simulink model "ASM1"  (R2024b)
settings: Solver=VariableStepAuto  StartTime=0.0  StopTime=100  RelTol=1e-2
values from neighbouring files (symbols this model uses):
  b_A = 0.05    [Input.m]
  b_H = 0.3    [Input.m]
  f_P = 0.08    [Input.m]
  i_X_B = 0.086    [Input.m]
  i_X_P = 0.06    [Input.m]
  k_a = 0.08    [Input.m]
  k_h = 3    [Input.m]
  K_N_H = 1    [Input.m]
  K_N_O = 0.5    [Input.m]
  K_O_A = 0.4    [Input.m]
  K_O_H = 0.2    [Input.m]
  K_S = 20    [Input.m]
  K_X = 0.03    [Input.m]
  mu_A = 0.8    [Input.m]
  mu_H = 6    [Input.m]
  nuy_g = 0.8    [Input.m]
  nuy_h = 0.4    [Input.m]
  Q_1 = 1000    [Input.m]
  Q_2 = Q_1    (= 1000)    [Input.m]
  S_ALK = 5    [Input.m]
  S_I = 40    [Input.m]
  S_ND = 8    [Input.m]
  S_NH = 1    [Input.m]
  S_NO = 0.5    [Input.m]
  S_O = 0.002    [Input.m]
  S_S = 125    [Input.m]
  V_tank = 10000    [Input.m]
  X_B_A = 1    [Input.m]
  X_B_H = 1    [Input.m]
  X_I = 100    [Input.m]
  X_ND = 10    [Input.m]
  X_P = 1    [Input.m]
  X_S = 250    [Input.m]
  Y_A = 0.24    [Input.m]
  Y_H = 0.67    [Input.m]
settings Model: Creator=luima  LastModifiedBy=luima

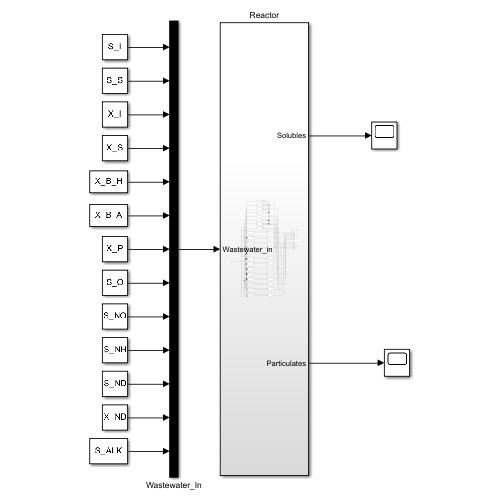
[thumbnail: Simulink's stored preview of the top-level diagram]
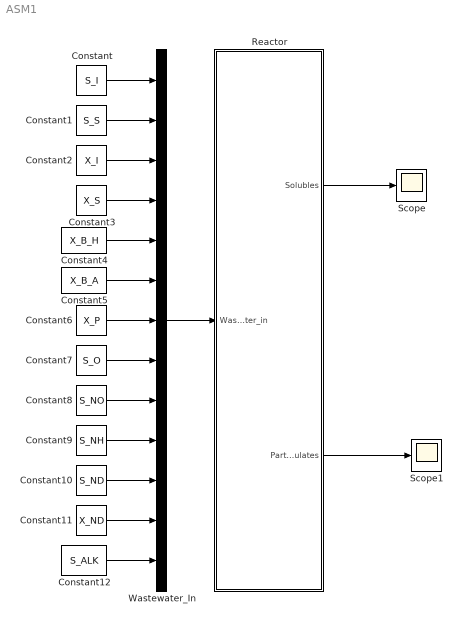
== system ASM1 ==
  Constant : Constant  Value=S_I
  Constant1 : Constant  Value=S_S
  Constant10 : Constant  Value=S_ND
  Constant11 : Constant  Value=X_ND
  Constant12 : Constant  Value=S_ALK
  Constant2 : Constant  Value=X_I
  Constant3 : Constant  Value=X_S
  Constant4 : Constant  Value=X_B_H
  Constant5 : Constant  Value=X_B_A
  Constant6 : Constant  Value=X_P
  Constant7 : Constant  Value=S_O
  Constant8 : Constant  Value=S_NO
  Constant9 : Constant  Value=S_NH
  Reactor : Subsystem
  Scope : Scope
  Scope1 : Scope
  Wastewater_In : Mux  Inputs=13
  wires:
  Constant/1 -> Wastewater_In/1
  Constant1/1 -> Wastewater_In/2
  Constant7/1 -> Wastewater_In/8
  Constant8/1 -> Wastewater_In/9
  Constant9/1 -> Wastewater_In/10
  Constant10/1 -> Wastewater_In/11
  Constant12/1 -> Wastewater_In/13
  Reactor/1(Solubles) -> Scope/1
  Reactor/2(Particulates) -> Scope1/1
  Constant2/1 -> Wastewater_In/3
  Constant3/1 -> Wastewater_In/4
  Constant4/1 -> Wastewater_In/5
  Constant5/1 -> Wastewater_In/6
  Constant6/1 -> Wastewater_In/7
  Constant11/1 -> Wastewater_In/12
  Wastewater_In/1 -> Reactor/1(Wastewater_in)

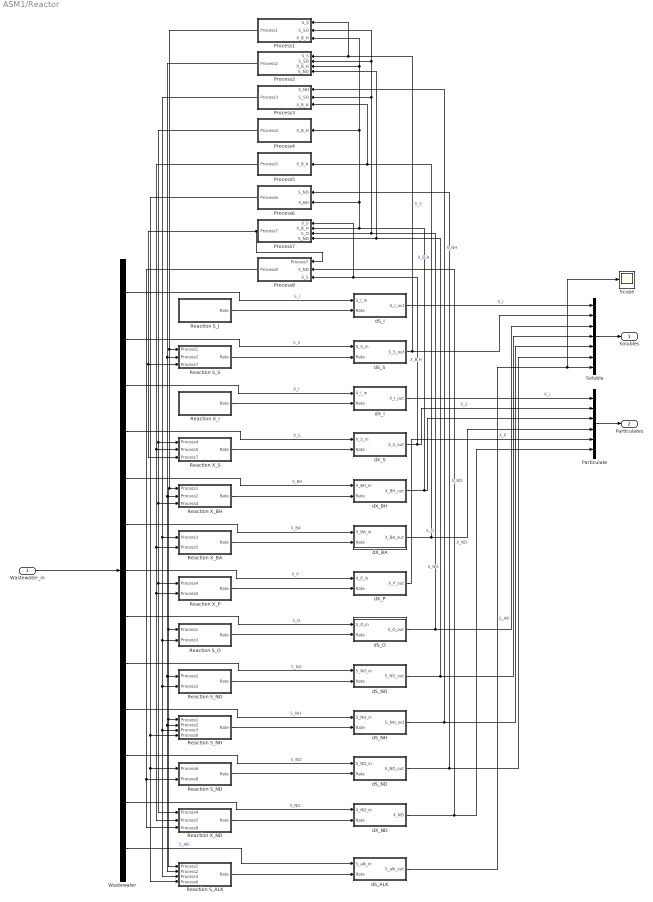
== system ASM1/Reactor ==
  Wastewater_in : Inport
  Particulate : Mux  Inputs=6
  Process1 : Subsystem
  Process2 : Subsystem
  Process3 : Subsystem
  Process4 : Subsystem
  Process5 : Subsystem
  Process6 : Subsystem
  Process7 : Subsystem
  Process8 : Subsystem
  Reaction S_ALK : Subsystem
  Reaction S_I : Subsystem
  Reaction S_ND : Subsystem
  Reaction S_NH : Subsystem
  Reaction S_NO : Subsystem
  Reaction S_O : Subsystem
  Reaction S_S : Subsystem
  Reaction X_BA : Subsystem
  Reaction X_BH : Subsystem
  Reaction X_I : Subsystem
  Reaction X_ND : Subsystem
  Reaction X_P : Subsystem
  Reaction X_S : Subsystem
  Scope : Scope
  Soluble : Mux  Inputs=7
  Wastewater : Demux  Outputs=13
  dS_ALK : Subsystem
  dS_I : Subsystem
  dS_ND : Subsystem
  dS_NH : Subsystem
  dS_NO : Subsystem
  dS_O : Subsystem
  dS_S : Subsystem
  dX_BA : Subsystem
  dX_BH : Subsystem
  dX_I : Subsystem
  dX_ND : Subsystem
  dX_P : Subsystem
  dX_S : Subsystem
  Solubles : Outport
  Particulates : Outport  Port=2
  wires:
  Process7/1(Process7) -> Process8/1(Process7), Reaction S_S/3(Process7), Reaction X_S/3(Process7)
  Process1/1(Process1) -> Reaction S_ALK/1(Process1), Reaction S_NH/1(Process1), Reaction S_O/1(Process1), Reaction X_BH/1(Process1), Reaction S_S/1(Process1)
  Process2/1(Process2) -> Reaction S_ALK/2(Process2), Reaction S_NH/2(Process2), Reaction S_NO/1(Process2), Reaction X_BH/2(Process2), Reaction S_S/2(Process2)
  Process3/1(Process3) -> Reaction X_BA/1(Process3), Reaction S_ALK/3(Process3), Reaction S_NH/3(Process3), Reaction S_NO/2(Process3), Reaction S_O/2(Process3)
  Process4/1(Process4) -> Reaction X_ND/1(Process4), Reaction X_P/1(Process4), Reaction X_BH/3(Process4), Reaction X_S/1(Process4)
  Process5/1(Process5) -> Reaction X_ND/2(Process5), Reaction X_P/2(Process5), Reaction X_BA/2(Process5), Reaction X_S/2(Process5)
  Process6/1(Process6) -> Reaction S_NH/4(Process6), Reaction S_ALK/4(Process6), Reaction S_ND/1(Process6)
  Process8/1(Process8) -> Reaction X_ND/3(Process8), Reaction S_ND/2(Process8)
  Reaction S_I/1(Rate) -> dS_I/2(Rate)
  dS_I/1(S_I_out) -> Soluble/1  "S_I"
  Wastewater/2 -> dS_S/1(S_S_in)  "S_S"
  dS_S/1(S_S_out) -> Process1/1(S_S), Process2/1(S_S), Soluble/2  "S_S"
  Reaction S_S/1(Rate) -> dS_S/2(Rate)
  Wastewater/3 -> dX_I/1(X_I_in)  "X_I"
  dX_I/1(X_I_out) -> Particulate/1  "X_I"
  Reaction X_I/1(Rate) -> dX_I/2(Rate)
  Wastewater/4 -> dX_S/1(X_S_in)  "X_S"
  dX_S/1(X_S_out) -> Process7/1(X_S), Process8/3(X_S), Particulate/2  "X_S"
  Reaction X_S/1(Rate) -> dX_S/2(Rate)
  Wastewater/5 -> dX_BH/1(X_BH_in)  "X_BH"
  Reaction X_BH/1(Rate) -> dX_BH/2(Rate)
  dX_BH/1(X_BH_out) -> Process1/3(X_B_H), Process2/3(X_B_H), Process4/1(X_B_H), Process6/2(X_BH), Process7/2(X_B_H), Particulate/3  "X_B,H"
  Wastewater/6 -> dX_BA/1(X_BA_in)  "X_BA"
  dX_BA/1(X_BA_out) -> Process3/3(X_B_A), Process5/1(X_B_A), Particulate/4  "X_B,A"
  Reaction X_BA/1(Rate) -> dX_BA/2(Rate)
  dX_P/1(X_P_out) -> Particulate/5  "X_P"
  Wastewater/7 -> dX_P/1(X_P_in)  "X_P"
  Reaction X_P/1(Rate) -> dX_P/2(Rate)
  Wastewater/8 -> dS_O/1(S_O_in)  "S_O"
  dS_O/1(S_O_out) -> Process1/2(S_SO), Process2/2(S_SO), Process3/2(S_SO), Process7/3(S_O), Soluble/3  "S_O"
  Reaction S_O/1(Rate) -> dS_O/2(Rate)
  Wastewater/9 -> dS_NO/1(S_NO_in)  "S_NO"
  dS_NO/1(S_NO_out) -> Process2/4(S_NO), Process7/4(S_NO), Soluble/4  "S_NO"
  Reaction S_NO/1(Rate) -> dS_NO/2(Rate)
  Wastewater/10 -> dS_NH/1(S_NH_in)  "S_NH"
  dS_NH/1(S_NH_out) -> Process3/1(S_NH), Soluble/5  "S_NH"
  Reaction S_NH/1(Rate) -> dS_NH/2(Rate)
  Wastewater/11 -> dS_ND/1(S_ND_in)  "S_ND"
  dS_ND/1(S_ND_out) -> Process6/1(S_ND), Soluble/6  "S_ND"
  Reaction S_ND/1(Rate) -> dS_ND/2(Rate)
  Wastewater/12 -> dX_ND/1(X_ND_in)  "X_ND"
  dX_ND/1(X_ND) -> Process8/2(X_ND), Particulate/6  "X_ND"
  Reaction X_ND/1(Rate) -> dX_ND/2(Rate)
  Wastewater/13 -> dS_ALK/1(S_alk_in)  "S_Alk"
  Reaction S_ALK/1(Rate) -> dS_ALK/2(Rate)
  dS_ALK/1(S_alk_out) -> Scope/1, Soluble/7  "S_Alk"
  Wastewater/1 -> dS_I/1(S_I_in)  "S_I"
  Soluble/1 -> Solubles/1
  Particulate/1 -> Particulates/1
  Wastewater_in/1 -> Wastewater/1

== system ASM1/Reactor/Process1 ==
  S_S : Inport
  S_SO : Inport  Port=2
  X_B_H : Inport  Port=3
  A/(A+B) : Subsystem
  A/(A+B)1 : Subsystem
  Constant : Constant  Value=mu_H
  Constant1 : Constant  Value=K_S
  Constant2 : Constant  Value=K_O_H
  Product : Product  Inputs=4
  Process1 : Outport
  wires:
  S_S/1 -> A/(A+B)/1(A)
  Constant1/1 -> A/(A+B)/2(B)
  S_SO/1 -> A/(A+B)1/1(A)
  Constant2/1 -> A/(A+B)1/2(B)
  Constant/1 -> Product/1
  A/(A+B)/1(Out1) -> Product/2
  A/(A+B)1/1(Out1) -> Product/3
  X_B_H/1 -> Product/4
  Product/1 -> Process1/1

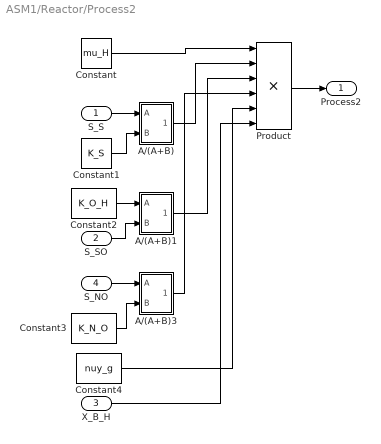
== system ASM1/Reactor/Process2 ==
  S_S : Inport
  S_SO : Inport  Port=2
  X_B_H : Inport  Port=3
  S_NO : Inport  Port=4
  A/(A+B) : Subsystem
  A/(A+B)1 : Subsystem
  A/(A+B)3 : Subsystem
  Constant : Constant  Value=mu_H
  Constant1 : Constant  Value=K_S
  Constant2 : Constant  Value=K_O_H
  Constant3 : Constant  Value=K_N_O
  Constant4 : Constant  Value=nuy_g
  Product : Product  Inputs=6
  Process2 : Outport
  wires:
  S_S/1 -> A/(A+B)/1(A)
  Constant1/1 -> A/(A+B)/2(B)
  Constant/1 -> Product/1
  A/(A+B)/1(Out1) -> Product/2
  A/(A+B)1/1(Out1) -> Product/3
  Constant2/1 -> A/(A+B)1/1(A)
  S_SO/1 -> A/(A+B)1/2(B)
  S_NO/1 -> A/(A+B)3/1(A)
  Constant3/1 -> A/(A+B)3/2(B)
  A/(A+B)3/1(Out1) -> Product/4
  Constant4/1 -> Product/5
  X_B_H/1 -> Product/6
  Product/1 -> Process2/1

== system ASM1/Reactor/Process3 ==
  S_NH : Inport
  S_SO : Inport  Port=2
  X_B_A : Inport  Port=3
  A/(A+B) : Subsystem
  A/(A+B)1 : Subsystem
  Constant : Constant  Value=mu_A
  Constant1 : Constant  Value=K_N_H
  Constant2 : Constant  Value=K_O_A
  Product : Product  Inputs=4
  Process3 : Outport
  wires:
  S_NH/1 -> A/(A+B)/1(A)
  Constant1/1 -> A/(A+B)/2(B)
  S_SO/1 -> A/(A+B)1/1(A)
  Constant2/1 -> A/(A+B)1/2(B)
  Constant/1 -> Product/1
  A/(A+B)/1(Out1) -> Product/2
  A/(A+B)1/1(Out1) -> Product/3
  X_B_A/1 -> Product/4
  Product/1 -> Process3/1

== system ASM1/Reactor/Process4 ==
  X_B_H : Inport
  Constant : Constant  Value=b_H
  Product : Product
  Process4 : Outport
  wires:
  Product/1 -> Process4/1
  Constant/1 -> Product/1
  X_B_H/1 -> Product/2

== system ASM1/Reactor/Process5 ==
  X_B_A : Inport
  Constant : Constant  Value=b_A
  Product : Product
  Process5 : Outport
  wires:
  Product/1 -> Process5/1
  Constant/1 -> Product/1
  X_B_A/1 -> Product/2

== system ASM1/Reactor/Process6 ==
  S_ND : Inport
  X_BH : Inport  Port=2
  Constant : Constant  Value=k_a
  Product : Product  Inputs=3
  Process6 : Outport
  wires:
  Product/1 -> Process6/1
  Constant/1 -> Product/1
  S_ND/1 -> Product/2
  X_BH/1 -> Product/3

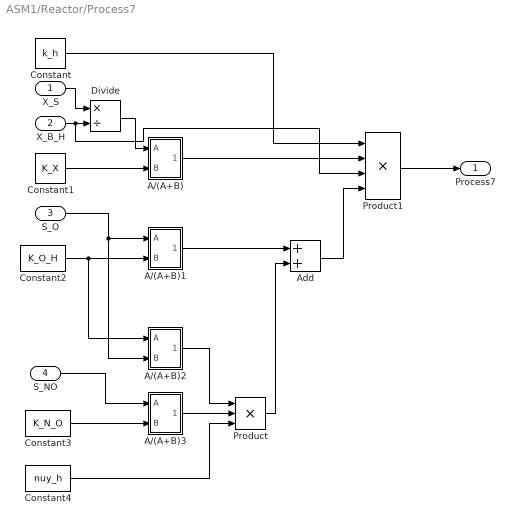
== system ASM1/Reactor/Process7 ==
  X_S : Inport
  X_B_H : Inport  Port=2
  S_O : Inport  Port=3
  S_NO : Inport  Port=4
  A/(A+B) : Subsystem
  A/(A+B)1 : Subsystem
  A/(A+B)2 : Subsystem
  A/(A+B)3 : Subsystem
  Add : Sum
  Constant : Constant  Value=k_h
  Constant1 : Constant  Value=K_X
  Constant2 : Constant  Value=K_O_H
  Constant3 : Constant  Value=K_N_O
  Constant4 : Constant  Value=nuy_h
  Divide : Product  Inputs=*/
  Product : Product  Inputs=3
  Product1 : Product  Inputs=4
  Process7 : Outport
  wires:
  X_S/1 -> Divide/1
  Constant1/1 -> A/(A+B)/2(B)
  Divide/1 -> A/(A+B)/1(A)
  Constant2/1 -> A/(A+B)2/1(A), A/(A+B)1/2(B)
  S_O/1 -> A/(A+B)2/2(B), A/(A+B)1/1(A)
  Constant3/1 -> A/(A+B)3/2(B)
  S_NO/1 -> A/(A+B)3/1(A)
  A/(A+B)3/1(Out1) -> Product/2
  Constant4/1 -> Product/3
  A/(A+B)2/1(Out1) -> Product/1
  Product/1 -> Add/2
  A/(A+B)1/1(Out1) -> Add/1
  Constant/1 -> Product1/1
  A/(A+B)/1(Out1) -> Product1/2
  Add/1 -> Product1/4
  Product1/1 -> Process7/1
  X_B_H/1 -> Product1/3, Divide/2

== system ASM1/Reactor/Process8 ==
  Process7 : Inport
  X_ND : Inport  Port=2
  X_S : Inport  Port=3
  Divide : Product  Inputs=**
  Divide1 : Product  Inputs=*/
  Process8 : Outport
  wires:
  X_ND/1 -> Divide1/1
  X_S/1 -> Divide1/2
  Divide1/1 -> Divide/2
  Process7/1 -> Divide/1
  Divide/1 -> Process8/1

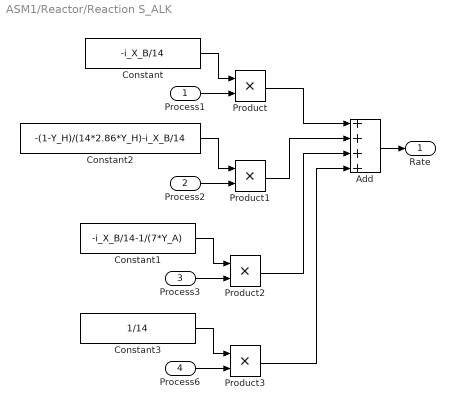
== system ASM1/Reactor/Reaction S_ALK ==
  Process1 : Inport
  Process2 : Inport  Port=2
  Process3 : Inport  Port=3
  Process6 : Inport  Port=4
  Add : Sum  Inputs=++++
  Constant : Constant  Value=-i_X_B/14
  Constant1 : Constant  Value=-i_X_B/14-1/(7*Y_A)
  Constant2 : Constant  Value=-(1-Y_H)/(14*2.86*Y_H)-i_X_B/14
  Constant3 : Constant  Value=1/14
  Product{,1..3} (4 alike) : Product
  Rate : Outport
  wires:
  Process1/1 -> Product/2
  Constant/1 -> Product/1
  Process2/1 -> Product1/2
  Constant2/1 -> Product1/1
  Product/1 -> Add/1
  Product1/1 -> Add/2
  Add/1 -> Rate/1
  Constant1/1 -> Product2/1
  Product2/1 -> Add/3
  Process3/1 -> Product2/2
  Process6/1 -> Product3/2
  Product3/1 -> Add/4
  Constant3/1 -> Product3/1

== system ASM1/Reactor/Reaction S_I ==
  Constant : Constant  Value=0
  Rate : Outport
  wires:
  Constant/1 -> Rate/1

== system ASM1/Reactor/Reaction S_ND ==
  Process6 : Inport
  Process8 : Inport  Port=2
  Add : Sum  Inputs=-+
  Rate : Outport
  wires:
  Process8/1 -> Add/2
  Process6/1 -> Add/1
  Add/1 -> Rate/1

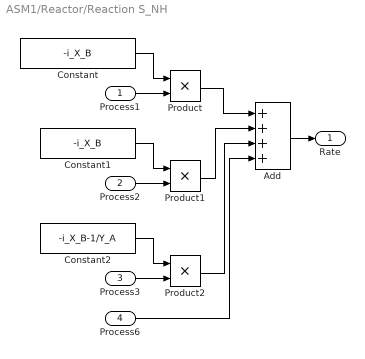
== system ASM1/Reactor/Reaction S_NH ==
  Process1 : Inport
  Process2 : Inport  Port=2
  Process3 : Inport  Port=3
  Process6 : Inport  Port=4
  Add : Sum  Inputs=++++
  Constant : Constant  Value=-i_X_B
  Constant1 : Constant  Value=-i_X_B
  Constant2 : Constant  Value=-i_X_B-1/Y_A
  Product : Product
  Product1 : Product
  Product2 : Product
  Rate : Outport
  wires:
  Process1/1 -> Product/2
  Constant/1 -> Product/1
  Process2/1 -> Product1/2
  Constant1/1 -> Product1/1
  Product/1 -> Add/1
  Product1/1 -> Add/2
  Add/1 -> Rate/1
  Process3/1 -> Product2/2
  Constant2/1 -> Product2/1
  Product2/1 -> Add/3
  Process6/1 -> Add/4

== system ASM1/Reactor/Reaction S_NO ==
  Process2 : Inport
  Process3 : Inport  Port=2
  Add : Sum
  Constant : Constant  Value=-(1-Y_H)/(2.86*Y_H)
  Constant1 : Constant  Value=1/Y_A
  Product : Product
  Product1 : Product
  Rate : Outport
  wires:
  Process2/1 -> Product/2
  Constant/1 -> Product/1
  Process3/1 -> Product1/2
  Constant1/1 -> Product1/1
  Product/1 -> Add/1
  Product1/1 -> Add/2
  Add/1 -> Rate/1

== system ASM1/Reactor/Reaction S_O ==
  Process1 : Inport
  Process3 : Inport  Port=2
  Add : Sum
  Constant : Constant  Value=-(1-Y_H)/Y_H
  Constant1 : Constant  Value=-(4.57-Y_A)/Y_A
  Product : Product
  Product1 : Product
  Rate : Outport
  wires:
  Process1/1 -> Product/2
  Constant/1 -> Product/1
  Process3/1 -> Product1/2
  Constant1/1 -> Product1/1
  Product/1 -> Add/1
  Product1/1 -> Add/2
  Add/1 -> Rate/1

== system ASM1/Reactor/Reaction S_S ==
  Process1 : Inport
  Process2 : Inport  Port=2
  Process7 : Inport  Port=3
  Add : Sum  Inputs=--
  Add1 : Sum
  Constant : Constant  Value=Y_H
  Divide : Product  Inputs=*/
  Rate : Outport
  wires:
  Process1/1 -> Add/1
  Process2/1 -> Add/2
  Constant/1 -> Divide/2
  Add/1 -> Divide/1
  Process7/1 -> Add1/2
  Divide/1 -> Add1/1
  Add1/1 -> Rate/1

== system ASM1/Reactor/Reaction X_BA ==
  Process3 : Inport
  Process5 : Inport  Port=2
  Add : Sum  Inputs=+-
  Rate : Outport
  wires:
  Process5/1 -> Add/2
  Process3/1 -> Add/1
  Add/1 -> Rate/1

== system ASM1/Reactor/Reaction X_BH ==
  Process1 : Inport
  Process2 : Inport  Port=2
  Process4 : Inport  Port=3
  Add : Sum  Inputs=++-
  Rate : Outport
  wires:
  Process2/1 -> Add/2
  Process1/1 -> Add/1
  Process4/1 -> Add/3
  Add/1 -> Rate/1

== system ASM1/Reactor/Reaction X_I ==
  Constant : Constant  Value=0
  Rate : Outport
  wires:
  Constant/1 -> Rate/1

== system ASM1/Reactor/Reaction X_ND ==
  Process4 : Inport
  Process5 : Inport  Port=2
  Process8 : Inport  Port=3
  Add : Sum  Inputs=++-
  Constant : Constant  Value=i_X_B-f_P*i_X_P
  Constant2 : Constant  Value=i_X_B-f_P*i_X_P
  Product : Product
  Product1 : Product
  Rate : Outport
  wires:
  Process4/1 -> Product/2
  Constant/1 -> Product/1
  Process5/1 -> Product1/2
  Constant2/1 -> Product1/1
  Product/1 -> Add/1
  Product1/1 -> Add/2
  Add/1 -> Rate/1
  Process8/1 -> Add/3

== system ASM1/Reactor/Reaction X_P ==
  Process4 : Inport
  Process5 : Inport  Port=2
  Add : Sum
  Constant : Constant  Value=f_P
  Product : Product
  Rate : Outport
  wires:
  Process5/1 -> Add/2
  Process4/1 -> Add/1
  Constant/1 -> Product/2
  Add/1 -> Product/1
  Product/1 -> Rate/1

== system ASM1/Reactor/Reaction X_S ==
  Process4 : Inport
  Process5 : Inport  Port=2
  Process7 : Inport  Port=3
  Add : Sum
  Constant : Constant  Value=1-f_P
  Product : Product
  Subtract : Sum  Inputs=+-
  Rate : Outport
  wires:
  Process5/1 -> Add/2
  Process4/1 -> Add/1
  Constant/1 -> Product/2
  Add/1 -> Product/1
  Process7/1 -> Subtract/2
  Product/1 -> Subtract/1
  Subtract/1 -> Rate/1

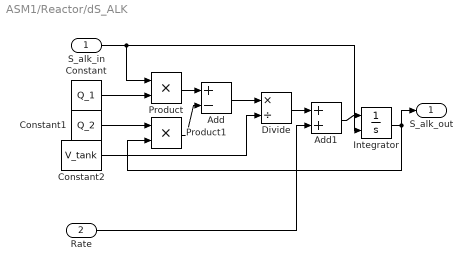
== system ASM1/Reactor/dS_ALK ==
  S_alk_in : Inport
  Rate : Inport  Port=2
  Add : Sum  Inputs=+-
  Add1 : Sum
  Constant : Constant  Value=Q_1
  Constant1 : Constant  Value=Q_2
  Constant2 : Constant  Value=V_tank
  Divide : Product  Inputs=*/
  Integrator : Integrator  InitialConditionSource=external
  Product : Product
  Product1 : Product
  S_alk_out : Outport
  wires:
  Constant/1 -> Product/2
  S_alk_in/1 -> Integrator/2, Product/1
  Integrator/1 -> S_alk_out/1, Product1/2
  Constant1/1 -> Product1/1
  Product/1 -> Add/1
  Product1/1 -> Add/2
  Constant2/1 -> Divide/2
  Add/1 -> Divide/1
  Rate/1 -> Add1/2
  Add1/1 -> Integrator/1
  Divide/1 -> Add1/1

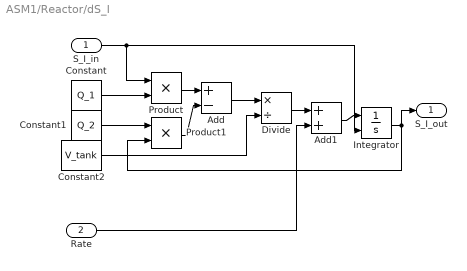
== system ASM1/Reactor/dS_I ==
  S_I_in : Inport
  Rate : Inport  Port=2
  Add : Sum  Inputs=+-
  Add1 : Sum
  Constant : Constant  Value=Q_1
  Constant1 : Constant  Value=Q_2
  Constant2 : Constant  Value=V_tank
  Divide : Product  Inputs=*/
  Integrator : Integrator  InitialConditionSource=external
  Product : Product
  Product1 : Product
  S_I_out : Outport
  wires:
  Constant/1 -> Product/2
  S_I_in/1 -> Integrator/2, Product/1
  Integrator/1 -> S_I_out/1, Product1/2
  Constant1/1 -> Product1/1
  Product/1 -> Add/1
  Product1/1 -> Add/2
  Constant2/1 -> Divide/2
  Add/1 -> Divide/1
  Add1/1 -> Integrator/1
  Divide/1 -> Add1/1
  Rate/1 -> Add1/2

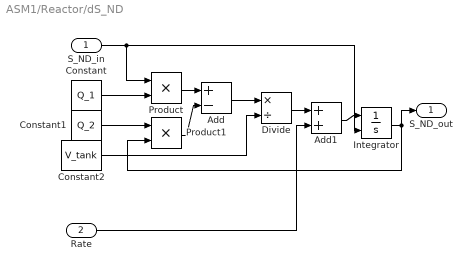
== system ASM1/Reactor/dS_ND ==
  S_ND_in : Inport
  Rate : Inport  Port=2
  Add : Sum  Inputs=+-
  Add1 : Sum
  Constant : Constant  Value=Q_1
  Constant1 : Constant  Value=Q_2
  Constant2 : Constant  Value=V_tank
  Divide : Product  Inputs=*/
  Integrator : Integrator  InitialConditionSource=external
  Product : Product
  Product1 : Product
  S_ND_out : Outport
  wires:
  Constant/1 -> Product/2
  S_ND_in/1 -> Integrator/2, Product/1
  Integrator/1 -> S_ND_out/1, Product1/2
  Constant1/1 -> Product1/1
  Product/1 -> Add/1
  Product1/1 -> Add/2
  Constant2/1 -> Divide/2
  Add/1 -> Divide/1
  Rate/1 -> Add1/2
  Add1/1 -> Integrator/1
  Divide/1 -> Add1/1

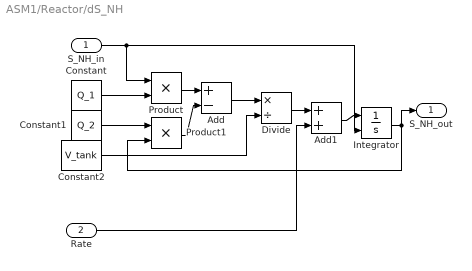
== system ASM1/Reactor/dS_NH ==
  S_NH_in : Inport
  Rate : Inport  Port=2
  Add : Sum  Inputs=+-
  Add1 : Sum
  Constant : Constant  Value=Q_1
  Constant1 : Constant  Value=Q_2
  Constant2 : Constant  Value=V_tank
  Divide : Product  Inputs=*/
  Integrator : Integrator  InitialConditionSource=external
  Product : Product
  Product1 : Product
  S_NH_out : Outport
  wires:
  Constant/1 -> Product/2
  S_NH_in/1 -> Integrator/2, Product/1
  Integrator/1 -> S_NH_out/1, Product1/2
  Constant1/1 -> Product1/1
  Product/1 -> Add/1
  Product1/1 -> Add/2
  Constant2/1 -> Divide/2
  Add/1 -> Divide/1
  Rate/1 -> Add1/2
  Add1/1 -> Integrator/1
  Divide/1 -> Add1/1

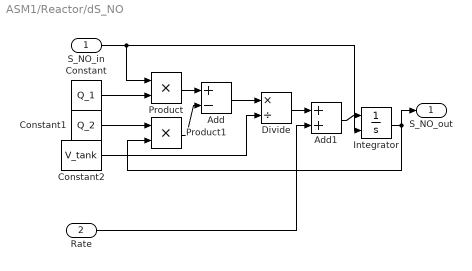
== system ASM1/Reactor/dS_NO ==
  S_NO_in : Inport
  Rate : Inport  Port=2
  Add : Sum  Inputs=+-
  Add1 : Sum
  Constant : Constant  Value=Q_1
  Constant1 : Constant  Value=Q_2
  Constant2 : Constant  Value=V_tank
  Divide : Product  Inputs=*/
  Integrator : Integrator  InitialConditionSource=external
  Product : Product
  Product1 : Product
  S_NO_out : Outport
  wires:
  Constant/1 -> Product/2
  S_NO_in/1 -> Integrator/2, Product/1
  Integrator/1 -> S_NO_out/1, Product1/2
  Constant1/1 -> Product1/1
  Product/1 -> Add/1
  Product1/1 -> Add/2
  Constant2/1 -> Divide/2
  Add/1 -> Divide/1
  Rate/1 -> Add1/2
  Add1/1 -> Integrator/1
  Divide/1 -> Add1/1

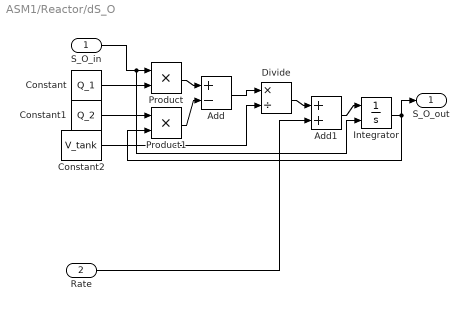
== system ASM1/Reactor/dS_O ==
  S_O_in : Inport
  Rate : Inport  Port=2
  Add : Sum  Inputs=+-
  Add1 : Sum
  Constant : Constant  Value=Q_1
  Constant1 : Constant  Value=Q_2
  Constant2 : Constant  Value=V_tank
  Divide : Product  Inputs=*/
  Integrator : Integrator  InitialConditionSource=external
  Product : Product
  Product1 : Product
  S_O_out : Outport
  wires:
  Constant/1 -> Product/2
  Integrator/1 -> S_O_out/1, Product1/2
  Constant1/1 -> Product1/1
  Product/1 -> Add/1
  Product1/1 -> Add/2
  Constant2/1 -> Divide/2
  Add/1 -> Divide/1
  Rate/1 -> Add1/2
  Add1/1 -> Integrator/1
  Divide/1 -> Add1/1
  S_O_in/1 -> Integrator/2, Product/1

== system ASM1/Reactor/dS_S ==
  S_S_in : Inport
  Rate : Inport  Port=2
  Add : Sum  Inputs=+-
  Add1 : Sum
  Constant : Constant  Value=Q_1
  Constant1 : Constant  Value=Q_2
  Constant2 : Constant  Value=V_tank
  Divide : Product  Inputs=*/
  Integrator : Integrator  InitialConditionSource=external
  Product : Product
  Product1 : Product
  S_S_out : Outport
  wires:
  Constant/1 -> Product/2
  S_S_in/1 -> Integrator/2, Product/1
  Integrator/1 -> S_S_out/1, Product1/2
  Constant1/1 -> Product1/1
  Product/1 -> Add/1
  Product1/1 -> Add/2
  Constant2/1 -> Divide/2
  Add/1 -> Divide/1
  Rate/1 -> Add1/2
  Add1/1 -> Integrator/1
  Divide/1 -> Add1/1

== system ASM1/Reactor/dX_BA ==
  X_BA_in : Inport
  Rate : Inport  Port=2
  Add : Sum  Inputs=+-
  Add1 : Sum
  Constant : Constant  Value=Q_1
  Constant1 : Constant  Value=Q_2
  Constant2 : Constant  Value=V_tank
  Divide : Product  Inputs=*/
  Integrator : Integrator  InitialConditionSource=external
  Product : Product
  Product1 : Product
  X_BA_out : Outport
  wires:
  Constant/1 -> Product/2
  X_BA_in/1 -> Integrator/2, Product/1
  Integrator/1 -> X_BA_out/1, Product1/2
  Constant1/1 -> Product1/1
  Product/1 -> Add/1
  Product1/1 -> Add/2
  Constant2/1 -> Divide/2
  Add/1 -> Divide/1
  Rate/1 -> Add1/2
  Add1/1 -> Integrator/1
  Divide/1 -> Add1/1

== system ASM1/Reactor/dX_BH ==
  X_BH_in : Inport
  Rate : Inport  Port=2
  Add : Sum  Inputs=+-
  Add1 : Sum
  Constant : Constant  Value=Q_1
  Constant1 : Constant  Value=Q_2
  Constant2 : Constant  Value=V_tank
  Divide : Product  Inputs=*/
  Integrator : Integrator  InitialConditionSource=external
  Product : Product
  Product1 : Product
  X_BH_out : Outport
  wires:
  Constant/1 -> Product/2
  X_BH_in/1 -> Integrator/2, Product/1
  Integrator/1 -> X_BH_out/1, Product1/2
  Constant1/1 -> Product1/1
  Product/1 -> Add/1
  Product1/1 -> Add/2
  Constant2/1 -> Divide/2
  Add/1 -> Divide/1
  Rate/1 -> Add1/2
  Add1/1 -> Integrator/1
  Divide/1 -> Add1/1

== system ASM1/Reactor/dX_I ==
  X_I_in : Inport
  Rate : Inport  Port=2
  Add : Sum  Inputs=+-
  Add1 : Sum
  Constant : Constant  Value=Q_1
  Constant1 : Constant  Value=Q_2
  Constant2 : Constant  Value=V_tank
  Divide : Product  Inputs=*/
  Integrator : Integrator  InitialConditionSource=external
  Product : Product
  Product1 : Product
  X_I_out : Outport
  wires:
  Constant/1 -> Product/2
  X_I_in/1 -> Integrator/2, Product/1
  Integrator/1 -> X_I_out/1, Product1/2
  Constant1/1 -> Product1/1
  Product/1 -> Add/1
  Product1/1 -> Add/2
  Constant2/1 -> Divide/2
  Add/1 -> Divide/1
  Rate/1 -> Add1/2
  Add1/1 -> Integrator/1
  Divide/1 -> Add1/1

== system ASM1/Reactor/dX_ND ==
  X_ND_in : Inport
  Rate : Inport  Port=2
  Add : Sum  Inputs=+-
  Add1 : Sum
  Constant : Constant  Value=Q_1
  Constant1 : Constant  Value=Q_2
  Constant2 : Constant  Value=V_tank
  Divide : Product  Inputs=*/
  Integrator : Integrator  InitialConditionSource=external
  Product : Product
  Product1 : Product
  X_ND : Outport
  wires:
  Constant/1 -> Product/2
  X_ND_in/1 -> Integrator/2, Product/1
  Integrator/1 -> X_ND/1, Product1/2
  Constant1/1 -> Product1/1
  Product/1 -> Add/1
  Product1/1 -> Add/2
  Constant2/1 -> Divide/2
  Add/1 -> Divide/1
  Rate/1 -> Add1/2
  Add1/1 -> Integrator/1
  Divide/1 -> Add1/1

== system ASM1/Reactor/dX_P ==
  X_P_in : Inport
  Rate : Inport  Port=2
  Add : Sum  Inputs=+-
  Add1 : Sum
  Constant : Constant  Value=Q_1
  Constant1 : Constant  Value=Q_2
  Constant2 : Constant  Value=V_tank
  Divide : Product  Inputs=*/
  Integrator : Integrator  InitialConditionSource=external
  Product : Product
  Product1 : Product
  X_P_out : Outport
  wires:
  Constant/1 -> Product/2
  X_P_in/1 -> Integrator/2, Product/1
  Integrator/1 -> X_P_out/1, Product1/2
  Constant1/1 -> Product1/1
  Product/1 -> Add/1
  Product1/1 -> Add/2
  Constant2/1 -> Divide/2
  Add/1 -> Divide/1
  Rate/1 -> Add1/2
  Add1/1 -> Integrator/1
  Divide/1 -> Add1/1

== system ASM1/Reactor/dX_S ==
  X_S_in : Inport
  Rate : Inport  Port=2
  Add : Sum  Inputs=+-
  Add1 : Sum  Inputs=+-
  Constant : Constant  Value=Q_1
  Constant1 : Constant  Value=Q_2
  Constant2 : Constant  Value=V_tank
  Divide : Product  Inputs=*/
  Integrator : Integrator  InitialConditionSource=external
  Product : Product
  Product1 : Product
  X_S_out : Outport
  wires:
  Constant/1 -> Product/2
  X_S_in/1 -> Integrator/2, Product/1
  Integrator/1 -> X_S_out/1, Product1/2
  Constant1/1 -> Product1/1
  Product/1 -> Add/1
  Product1/1 -> Add/2
  Constant2/1 -> Divide/2
  Add/1 -> Divide/1
  Add1/1 -> Integrator/1
  Divide/1 -> Add1/1
  Rate/1 -> Add1/2

== system ASM1/Reactor/Process1/A//(A+B) ==
  A : Inport
  B : Inport  Port=2
  Add : Sum
  Divide : Product  Inputs=*/
  Out1 : Outport
  wires:
  B/1 -> Add/2
  A/1 -> Divide/1, Add/1
  Divide/1 -> Out1/1
  Add/1 -> Divide/2

== system ASM1/Reactor/Process1/A//(A+B)1 ==
  A : Inport
  B : Inport  Port=2
  Add : Sum
  Divide : Product  Inputs=*/
  Out1 : Outport
  wires:
  B/1 -> Add/2
  A/1 -> Divide/1, Add/1
  Divide/1 -> Out1/1
  Add/1 -> Divide/2

== system ASM1/Reactor/Process2/A//(A+B) ==
  A : Inport
  B : Inport  Port=2
  Add : Sum
  Divide : Product  Inputs=*/
  Out1 : Outport
  wires:
  B/1 -> Add/2
  A/1 -> Divide/1, Add/1
  Divide/1 -> Out1/1
  Add/1 -> Divide/2

== system ASM1/Reactor/Process2/A//(A+B)1 ==
  A : Inport
  B : Inport  Port=2
  Add : Sum
  Divide : Product  Inputs=*/
  Out1 : Outport
  wires:
  B/1 -> Add/2
  A/1 -> Divide/1, Add/1
  Divide/1 -> Out1/1
  Add/1 -> Divide/2

== system ASM1/Reactor/Process2/A//(A+B)3 ==
  A : Inport
  B : Inport  Port=2
  Add : Sum
  Divide : Product  Inputs=*/
  Out1 : Outport
  wires:
  B/1 -> Add/2
  A/1 -> Divide/1, Add/1
  Divide/1 -> Out1/1
  Add/1 -> Divide/2

== system ASM1/Reactor/Process3/A//(A+B) ==
  A : Inport
  B : Inport  Port=2
  Add : Sum
  Divide : Product  Inputs=*/
  Out1 : Outport
  wires:
  B/1 -> Add/2
  A/1 -> Divide/1, Add/1
  Divide/1 -> Out1/1
  Add/1 -> Divide/2

== system ASM1/Reactor/Process3/A//(A+B)1 ==
  A : Inport
  B : Inport  Port=2
  Add : Sum
  Divide : Product  Inputs=*/
  Out1 : Outport
  wires:
  B/1 -> Add/2
  A/1 -> Divide/1, Add/1
  Divide/1 -> Out1/1
  Add/1 -> Divide/2

== system ASM1/Reactor/Process7/A//(A+B) ==
  A : Inport
  B : Inport  Port=2
  Add : Sum
  Divide : Product  Inputs=*/
  Out1 : Outport
  wires:
  B/1 -> Add/2
  A/1 -> Divide/1, Add/1
  Divide/1 -> Out1/1
  Add/1 -> Divide/2

== system ASM1/Reactor/Process7/A//(A+B)1 ==
  A : Inport
  B : Inport  Port=2
  Add : Sum
  Divide : Product  Inputs=*/
  Out1 : Outport
  wires:
  B/1 -> Add/2
  A/1 -> Divide/1, Add/1
  Divide/1 -> Out1/1
  Add/1 -> Divide/2

== system ASM1/Reactor/Process7/A//(A+B)2 ==
  A : Inport
  B : Inport  Port=2
  Add : Sum
  Divide : Product  Inputs=*/
  Out1 : Outport
  wires:
  B/1 -> Add/2
  A/1 -> Divide/1, Add/1
  Divide/1 -> Out1/1
  Add/1 -> Divide/2

== system ASM1/Reactor/Process7/A//(A+B)3 ==
  A : Inport
  B : Inport  Port=2
  Add : Sum
  Divide : Product  Inputs=*/
  Out1 : Outport
  wires:
  B/1 -> Add/2
  A/1 -> Divide/1, Add/1
  Divide/1 -> Out1/1
  Add/1 -> Divide/2
